simulink model "USAResseCascata"  (R2017a)
settings: Solver=VariableStepAuto  StartTime=0.0  StopTime=50  RelTol=1e-3
settings Model: Creator=julia  LastModifiedBy=julia

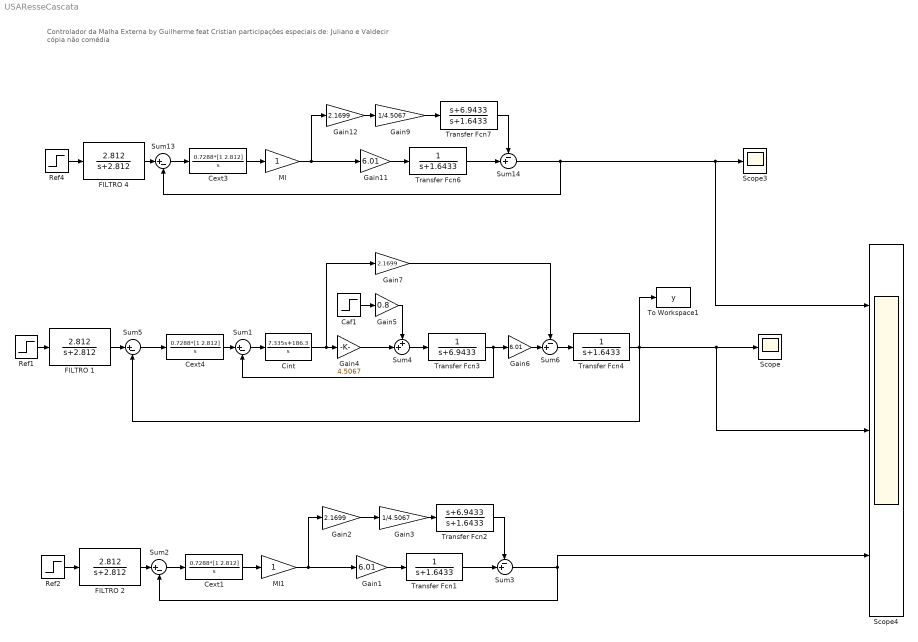
== system USAResseCascata ==
  note: Controlador da Malha Externa by Guilherme feat Cristian
      | participações especiais de: Juliano e Valdecir
      | cópia não comédia
  Caf1 : Step  Time=20  After=0.05  SampleTime=0
  Cext1 : TransferFcn  Numerator=0.7288*[1 2.812]  Denominator=[1 0]
  Cext3 : TransferFcn  Numerator=0.7288*[1 2.812]  Denominator=[1 0]
  Cext4 : TransferFcn  Numerator=0.7288*[1 2.812]  Denominator=[1 0]
  Cint : TransferFcn  Numerator=[7.335 186.3]  Denominator=[1 0]
  FILTRO 1 : TransferFcn  Numerator=[2.812]  Denominator=[1 2.812]
  FILTRO 2 : TransferFcn  Numerator=[2.812]  Denominator=[1 2.812]
  FILTRO 4 : TransferFcn  Numerator=[2.812]  Denominator=[1 2.812]
  Gain1 : Gain  Gain=6.01
  Gain11 : Gain  Gain=6.01
  Gain12 : Gain  Gain=2.1699
  Gain2 : Gain  Gain=2.1699
  Gain3 : Gain  Gain=1/4.5067
  Gain4 : Gain  Gain=4.5067
  Gain5 : Gain  Gain=0.8
  Gain6 : Gain  Gain=6.01
  Gain7 : Gain  Gain=2.1699
  Gain9 : Gain  Gain=1/4.5067
  MI : Gain
  MI1 : Gain
  Ref1 : Step  Time=0  After=0.1  SampleTime=0
  Ref2 : Step  Time=0  After=0.1  SampleTime=0
  Ref4 : Step  Time=0  After=0.1  SampleTime=0
  Scope : Scope
  Scope3 : Scope
  Scope4 : Scope  NumInputPorts=3
  Sum{1..2,5,13} (4 alike) : Sum  Inputs=|+-
  Sum14 : Sum  Inputs=-+|
  Sum3 : Sum  Inputs=-+|
  Sum4 : Sum  Inputs=++|
  Sum6 : Sum  Inputs=-+|
  To Workspace1 : ToWorkspace  VariableName=y  SaveFormat=Timeseries  SampleTime=-1
  Transfer Fcn1 : TransferFcn  Denominator=[1 1.6433]
  Transfer Fcn2 : TransferFcn  Numerator=[1 6.9433]  Denominator=[1 1.6433]
  Transfer Fcn3 : TransferFcn  Denominator=[1 6.9433]
  Transfer Fcn4 : TransferFcn  Denominator=[1 1.6433]
  Transfer Fcn6 : TransferFcn  Denominator=[1 1.6433]
  Transfer Fcn7 : TransferFcn  Numerator=[1 6.9433]  Denominator=[1 1.6433]
  wires:
  Caf1/1 -> Gain5/1
  Gain5/1 -> Sum4/1
  Transfer Fcn4/1 -> Scope4/2, Scope/1, To Workspace1/1, Sum5/2
  Sum4/1 -> Transfer Fcn3/1
  Transfer Fcn3/1 -> Gain6/1, Sum1/2
  Ref1/1 -> FILTRO 1/1
  FILTRO 1/1 -> Sum5/1
  Gain4/1 -> Sum4/2
  Sum5/1 -> Cext4/1
  Cext4/1 -> Sum1/1
  Sum1/1 -> Cint/1
  Cint/1 -> Gain7/1, Gain4/1
  Gain6/1 -> Sum6/2
  Sum6/1 -> Transfer Fcn4/1
  Gain7/1 -> Sum6/1
  Sum13/1 -> Cext3/1
  FILTRO 4/1 -> Sum13/1
  Ref4/1 -> FILTRO 4/1
  Cext3/1 -> MI/1
  Gain11/1 -> Transfer Fcn6/1
  Gain9/1 -> Transfer Fcn7/1
  Gain12/1 -> Gain9/1
  Transfer Fcn7/1 -> Sum14/1
  MI/1 -> Gain12/1, Gain11/1
  Sum14/1 -> Scope4/1, Scope3/1, Sum13/2
  Transfer Fcn6/1 -> Sum14/2
  Transfer Fcn1/1 -> Sum3/2
  Sum3/1 -> Scope4/3, Sum2/2
  MI1/1 -> Gain1/1, Gain2/1
  Gain2/1 -> Gain3/1
  Gain3/1 -> Transfer Fcn2/1
  Gain1/1 -> Transfer Fcn1/1
  Cext1/1 -> MI1/1
  Ref2/1 -> FILTRO 2/1
  FILTRO 2/1 -> Sum2/1
  Sum2/1 -> Cext1/1
  Transfer Fcn2/1 -> Sum3/1
